simulink model "EX21"  (R2013a)
settings: Solver=ode3  StartTime=0.0  StopTime=5e-3  FixedStep=1.25e-6  RelTol=1e-3
libraries: dsparch4 x1
settings Model: Creator=Dennis Silage  LastModifiedBy=Silage
settings DataIOCC: SignalLoggingSaveFormat=ModelDataLogs
settings OptimizationCC: ExpressionDepthLimit=2147483647  InitFltsAndDblsToZero=on
settings DebuggingCC: FcnCallInpInsideContextMsg=UseLocalSettings  StrictBusMsg=Warning
settings GRTTargetCC: CombineOutputUpdateFcns=off  GRTInterface=on

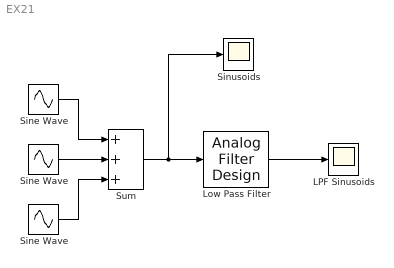
== system EX21 ==
  " Sine Wave " : Sin  Amplitude=0.2  Frequency=5000*pi  SampleTime=1.25e-6
  LPF Sinusoids : Scope
      settings: YMin=-1.5  YMax=1.5
  Low Pass Filter : dsparch4/Analog Filter Design  method=Butterworth  filttype=Lowpass  N=3  Wlo=pi*2500  Whi=80  Rp=2  Rs=40
  Sine Wave : Sin  Frequency=1000*pi  SampleTime=1.25e-6
  "Sine Wave " : Sin  Amplitude=0.5  Frequency=3000*pi  SampleTime=1.25e-6
  Sinusoids : Scope
  Sum : Sum  Inputs=+++
  wires:
  "Sine Wave "/1 -> Sum/2
  " Sine Wave "/1 -> Sum/3
  Sine Wave/1 -> Sum/1
  Sum/1 -> Sinusoids/1, Low Pass Filter/1
  Low Pass Filter/1 -> LPF Sinusoids/1
